simulink model "LinearToRotation"  (R2024b)
settings: Solver=VariableStepAuto  StartTime=0.0  StopTime=10.0  RelTol=1e-3
model workspace (MAT data in the model file):
  J_eq = 1
  L = 1
  Tc = 1
  b = 1
  efficiency = 1
settings Model: Creator=khalidwaleed  LastModifiedBy=khalidwaleed

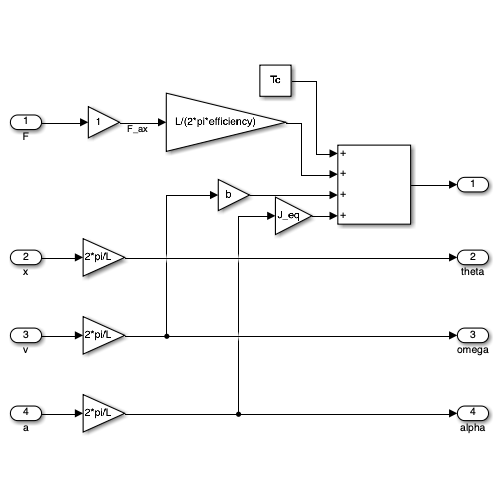
[thumbnail: Simulink's stored preview of the top-level diagram]
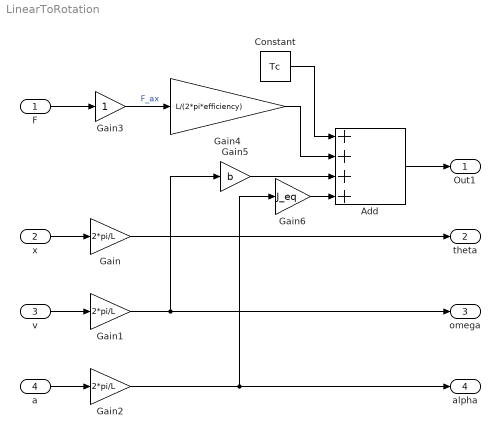
== system LinearToRotation ==
  F : Inport
  x : Inport  Port=2
  v : Inport  Port=3
  a : Inport  Port=4
  Add : Sum  Inputs=++++
  Constant : Constant  Value=Tc
  Gain : Gain  Gain=2*pi/L
  Gain1 : Gain  Gain=2*pi/L
  Gain2 : Gain  Gain=2*pi/L
  Gain3 : Gain
  Gain4 : Gain  Gain=L/(2*pi*efficiency)
  Gain5 : Gain  Gain=b
  Gain6 : Gain  Gain=J_eq
  Out1 : Outport
  theta : Outport  Port=2
  omega : Outport  Port=3
  alpha : Outport  Port=4
  wires:
  a/1 -> Gain2/1
  v/1 -> Gain1/1
  x/1 -> Gain/1
  Gain/1 -> theta/1
  Gain1/1 -> Gain5/1, omega/1
  Gain2/1 -> Gain6/1, alpha/1
  F/1 -> Gain3/1
  Gain3/1 -> Gain4/1  "F_ax"
  Add/1 -> Out1/1
  Gain5/1 -> Add/3
  Gain6/1 -> Add/4
  Constant/1 -> Add/1
  Gain4/1 -> Add/2
